simulink model "Scara"  (R2018a)
settings: Solver=ode1  StartTime=0.0  StopTime=Inf  FixedStep=0.001  RelTol=1e-3
PostLoadFcn:
  | , if any(exist('dsrtsu_mdlpostloadfcn', 'file') == [2, 3, 6]), try dsrtsu_mdlpostloadfcn('Execute', bdroot); catch fprintf('Error in PostLoadFcn (dsrtsu_mdlpostloadfcn) for model "%s":\n %s\n', bdroot, lasterr); end, end,
Description:
  | Standard RTI1007 template.
  | Supported MATLAB version:  R2018b.
settings Model: Tag=RTI1007  DSRTSU_INTERNAL_RTI_VER=530  DSRTSU_INTERNAL_RTI_TYPE=rti1007  RTICANMMDATA=struct('GeneralSetupData',struct('modelroot','Z:\public\Transfer\Mueller\DOB','generalsettings',struct('filesettings',struct('destfolder',struct('Name','RTICANMM_FILES','Check',1),'buildfolder',struct('Name','.','Check',1),'AbsDestfolder',struct('Name','Z:\public\Transfer\Mueller\DOB\RTICANMM_FILES'),'AbsBuildfolder',struct('Name','Z:\public\Transfer\Mueller\DOB'))),'options',struct('addpaths',1,'rmpaths',1,'addtrcexclusion',logical(1),'cannavigator',struct('checkmonitoring',0),'show_usrtrc',0,'use_usrtrc',0),'advanced',struct('options',ones(1,100)),'MPSetup',{{}},'RTI',struct('Type','RTI1007','Ver','7.11','Date','02-Nov-2018'),'modelname','plasticScara','block','plasticScara'))  DSRTSU_INTERNAL_RTIFPGA=120  Creator=User  LastModifiedBy=Müller
settings OptimizationCC: BlockReduction=off  OptimizeBlockIOStorage=off  BufferReuse=off  GlobalBufferReuse=off  ExpressionFolding=off  LocalBlockOutputs=off  OptimizeDataStoreBuffers=off  BusAssignmentInplaceUpdate=off
settings HardwareCC: ProdBitPerPointer=32  ProdBitPerSizeT=32  ProdBitPerPtrDiffT=32  ProdLargestAtomicInteger=Integer  ProdEndianess=BigEndian  ProdWordSize=32  ProdHWDeviceType=Custom Processor->Custom  TargetIntDivRoundTo=Zero  TargetEndianess=BigEndian  TargetHWDeviceType=Custom Processor->Custom
settings SFSimCC: MATLABDynamicMemAlloc=off
settings RTWCC: SystemTargetFile=rti1007.tlc  MakeCommand=make_rti  TemplateMakefile=rti1007.tmf  Description=dSPACE DS1007 Hardware Platform
settings CodeAppCC: StateflowObjectComments=on
settings STFCustomTargetCC: ParMdlRefBuildCompliant=on  MatFileLogging=on  GRTInterface=off  SystemTargetFile=rti1007.tlc
settings GRTTargetCC: TargetLangStandard=C89/C90 (ANSI)  CompOptLevelCompliant=off  ConcurrentExecutionCompliant=off  CombineOutputUpdateFcns=off  CPPClassGenCompliant=off  UseToolchainInfoCompliant=off
settings ConfigComp: CovMetricSettings=dswe

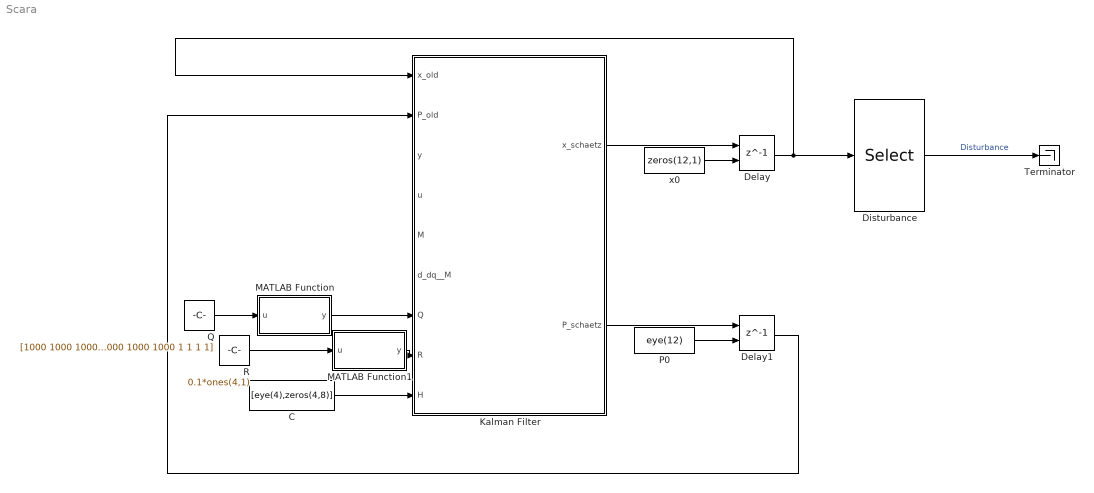
== system Scara ==
  C : Constant  Value=[eye(4),zeros(4,8)]
  Delay : Delay  DelayLength=1  InitialConditionSource=Input port
      settings: InputPortMap=u0,p4
  Delay1 : Delay  DelayLength=1  InitialConditionSource=Input port
      settings: InputPortMap=u0,p4
  Disturbance : Selector  InputPortWidth=12  IndexOptions=Index vector (dialog)  Indices=9:12  OutputSizes=1
  Kalman Filter : MATLAB Function  TreatAsAtomicUnit=on
  MATLAB Function : MATLAB Function  TreatAsAtomicUnit=on
  MATLAB Function1 : MATLAB Function  TreatAsAtomicUnit=on
  P0 : Constant  Value=eye(12)
  Q : Constant  Value=[1000 1000 1000 1000 1000 1000 1000 1000 1 1 1 1]
  R : Constant  Value=0.1*ones(4,1)
  Terminator : Terminator
  x0 : Constant  Value=zeros(12,1)
  wires:
  x0/1 -> Delay/2
  Delay1/1 -> Kalman Filter/2(P_old)
  P0/1 -> Delay1/2
  Kalman Filter/1(x_schaetz) -> Delay/1
  Kalman Filter/2(P_schaetz) -> Delay1/1
  Delay/1 -> Disturbance/1, Kalman Filter/1(x_old)
  MATLAB Function/1(y) -> Kalman Filter/7(Q)
  Q/1 -> MATLAB Function/1(u)
  MATLAB Function1/1(y) -> Kalman Filter/8(R)
  R/1 -> MATLAB Function1/1(u)
  C/1 -> Kalman Filter/9(H)
  Disturbance/1 -> Terminator/1  "Disturbance"

== matlab function Scara/MATLAB Function1 ==
  data: u input; y output
function y = makeDiag(u)

y = diag(u);

== matlab function Scara/MATLAB Function ==
  data: u input; y output
function y = makeDiag(u)

y = diag(u);

== matlab function Scara/Kalman Filter ==
  data: x_old input; P_old input; y input; u input; x_schaetz output; M input; d_dq__M input; Q input; R input; P_schaetz output; H input
function [x_schaetz,P_schaetz] = fcn(x_old,P_old,y,u,M,d_dq__M,Q,R,H)
%% @author daniel.mueller@isys.uni-stuttgart.de
% Inputs:   x_old - last step observer state
%            P_old - Covariance Noise
%            y - Measurement
%            u - Mechanical input, i.e. tau in the paper
%            M - Intertia matrix
%            d_dq__M - derivative of Intertia matrix
%            Q - System noise
%            R - Measurment noise
%            H - Derivative of the output equation h(x), note that it is
%                g(x) in the paper
% Implementation and convetnion of the EKF according to Wikipedia 
%                    (https://en.wikipedia.org/wiki/Extended_Kalman_filter)

% Sample time
dt = 1e-3; 
%System equation
f = [x_old(5:8);
    M\(u+x_old(9:12));
    zeros(4,1)];
%Derivative of System equation
F = zeros(12,12);
F_int = [eye(4),zeros(4,8);
    zeros(4), eye(4), zeros(4);
    zeros(4,8), eye(4)];
for ii = 1:4
    F(5:8,ii) = M\(d_dq__M(:,:,ii)/M)*((u+ x_old(9:12)));
end
F(5:8,9:12) = inv(M);
F(1:4,5:8) = eye(4);
F(:,:) = dt*(F(:,:))+F_int;

%% Prediction
x_pred =  x_old + dt*f;
P_pred = F*P_old*F' + Q;
%% Update
S = R + H*P_pred*H';
K = P_pred*H'/S;
P_schaetz = (eye(12)-K*H)*P_pred;
x_schaetz = x_pred + K*(y-H*x_pred);

end
